simulink model "Raider_test"  (R2016a)
settings: Solver=VariableStepAuto  StartTime=0.0  StopTime=inf  RelTol=1e-3
model workspace (MAT data in the model file):
  SL_ROS_VariableLengthArrays_MaxSizes.CommonInfo.ArrayTruncateAction = 'EmitWarning'
  SL_ROS_VariableLengthArrays_MaxSizes.MsgTypeMap = containers.Map
  SL_ROS_VariableLengthArrays_MaxSizes.MsgTypeMap.serialization.keys = {'sensor_msgs/Image', 'sensor_msgs/JointState'}
  SL_ROS_VariableLengthArrays_MaxSizes.MsgTypeMap.serialization.values{1}(1).PropertyName = 'Encoding'
  SL_ROS_VariableLengthArrays_MaxSizes.MsgTypeMap.serialization.values{1}(1).DataType = 'uint8'
  SL_ROS_VariableLengthArrays_MaxSizes.MsgTypeMap.serialization.values{1}(1).MaxLength = 128
  SL_ROS_VariableLengthArrays_MaxSizes.MsgTypeMap.serialization.values{1}(2).PropertyName = 'Data'
  SL_ROS_VariableLengthArrays_MaxSizes.MsgTypeMap.serialization.values{1}(2).DataType = 'uint8'
  SL_ROS_VariableLengthArrays_MaxSizes.MsgTypeMap.serialization.values{1}(2).MaxLength = 2000000
  SL_ROS_VariableLengthArrays_MaxSizes.MsgTypeMap.serialization.values{2}(1).PropertyName = 'Name'
  SL_ROS_VariableLengthArrays_MaxSizes.MsgTypeMap.serialization.values{2}(1).DataType = 'std_msgs/String'
  SL_ROS_VariableLengthArrays_MaxSizes.MsgTypeMap.serialization.values{2}(1).MaxLength = 20
  SL_ROS_VariableLengthArrays_MaxSizes.MsgTypeMap.serialization.values{2}(2).PropertyName = 'Position'
  SL_ROS_VariableLengthArrays_MaxSizes.MsgTypeMap.serialization.values{2}(2).DataType = 'double'
  SL_ROS_VariableLengthArrays_MaxSizes.MsgTypeMap.serialization.values{2}(2).MaxLength = 128
  SL_ROS_VariableLengthArrays_MaxSizes.MsgTypeMap.serialization.values{2}(3).PropertyName = 'Velocity'
  SL_ROS_VariableLengthArrays_MaxSizes.MsgTypeMap.serialization.values{2}(3).DataType = 'double'
  SL_ROS_VariableLengthArrays_MaxSizes.MsgTypeMap.serialization.values{2}(3).MaxLength = 128
  SL_ROS_VariableLengthArrays_MaxSizes.MsgTypeMap.serialization.values{2}(4).PropertyName = 'Effort'
  SL_ROS_VariableLengthArrays_MaxSizes.MsgTypeMap.serialization.values{2}(4).DataType = 'double'
  SL_ROS_VariableLengthArrays_MaxSizes.MsgTypeMap.serialization.values{2}(4).MaxLength = 128
  SL_ROS_VariableLengthArrays_MaxSizes.MsgTypeMap.serialization.uniformity = 0
  SL_ROS_VariableLengthArrays_MaxSizes.MsgTypeMap.serialization.keyType = 'char'
  SL_ROS_VariableLengthArrays_MaxSizes.MsgTypeMap.serialization.valueType = 'any'
libraries: robotlib x81
settings Model: Creator=xavidz  LastModifiedBy=xavidz
settings DataIOCC: LimitDataPoints=on
settings DebuggingCC: AllowSymbolicDim=off
settings ModelReferenceCC: PropagateSignalLabelsOutOfModel=off
settings GRTTargetCC: GeneratePreprocessorConditionals=Use local settings

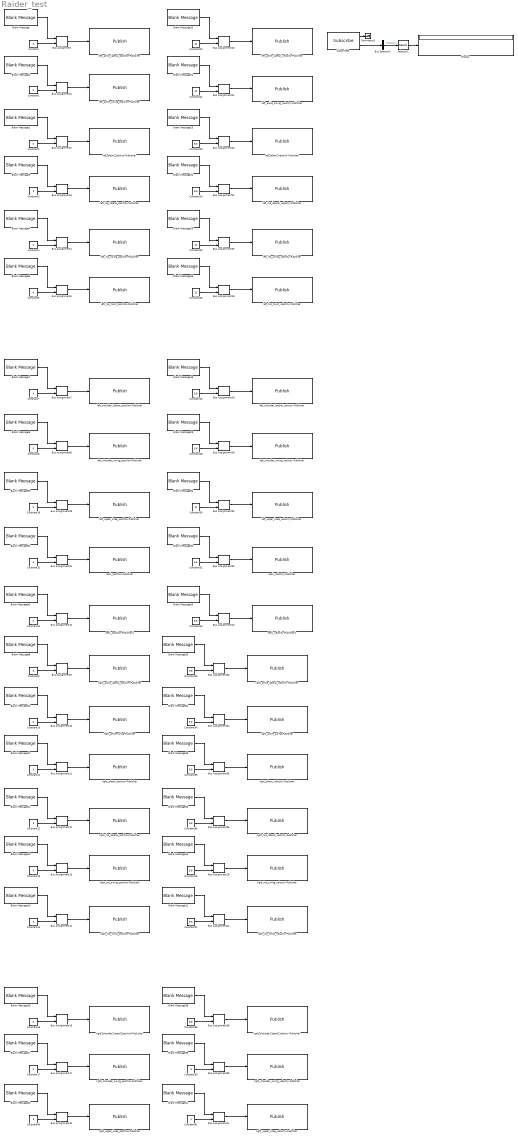
== system Raider_test ==
  Blank Message{,1..5,7..14,16..26,28..36,38..43} (40 alike) : robotlib/Blank Message  SourceLibraryInfo=This block requires Robotics System Toolbox  messageType=std_msgs/Float64  SampleTime=inf
  Bus Assignment{,1..5,7..14,16..26,28..36,38..43} (40 alike) : BusAssignment  AssignedSignals=Data
  Bus Selector3 : BusSelector  OutputSignals=Position
  Constant{,1..2,4..5,7..14,16..17,29,31,40,42} (19 alike) : Constant  Value=0
  Constant{18..19,21,23..24,28,32..36,38,43} (13 alike) : Constant  Value=5.6
  Constant{20,22,25..26,30} (5 alike) : Constant  Value=12
  Constant3 : Constant  Value=2
  Constant39 : Constant  Value=3
  Constant41 : Constant
  Display : Display
  Selector1 : Selector  IndexOptions=Select all  Indices=1  OutputSizes=1
  Subscribe3 : robotlib/Subscribe  SourceLibraryInfo=This block requires Robotics System Toolbox  topicSource=Select from ROS network  topic=/raider/joint_states  messageType=sensor_msgs/JointState  sampleTime=-1  messageQueueLength=1
  Terminator3 : Terminator
  left_ankle_lateral_position-Publisher : robotlib/Publish  SourceLibraryInfo=This block requires Robotics System Toolbox  topicSource=Select from ROS network  topic=/raider/l_ankle_lateral_position_controller/command  messageType=std_msgs/Float64  messageQueueLength=1
  left_ankle_lateral_velocity-Publisher : robotlib/Publish  SourceLibraryInfo=This block requires Robotics System Toolbox  topicSource=Select from ROS network  topic=/raider/l_ankle_lateral_velocity_controller/command  messageType=std_msgs/Float64  messageQueueLength=1
  left_ankle_swing_position-Publisher : robotlib/Publish  SourceLibraryInfo=This block requires Robotics System Toolbox  topicSource=Select from ROS network  topic=/raider/l_ankle_swing_position_controller/command  messageType=std_msgs/Float64  messageQueueLength=1
  left_ankle_swing_velocity-Publisher : robotlib/Publish  SourceLibraryInfo=This block requires Robotics System Toolbox  topicSource=Select from ROS network  topic=/raider/l_ankle_swing_velocity_controller/command  messageType=std_msgs/Float64  messageQueueLength=1
  left_elbow_position-Publisher : robotlib/Publish  SourceLibraryInfo=This block requires Robotics System Toolbox  topicSource=Select from ROS network  topic=/raider/l_elbow_position_controller/command  messageType=std_msgs/Float64  messageQueueLength=1
  left_elbow_velocity-Publisher : robotlib/Publish  SourceLibraryInfo=This block requires Robotics System Toolbox  topicSource=Select from ROS network  topic=/raider/l_elbow_velocity_controller/command  messageType=std_msgs/Float64  messageQueueLength=1
  left_hip_lateral_position-Publisher : robotlib/Publish  SourceLibraryInfo=This block requires Robotics System Toolbox  topicSource=Select from ROS network  topic=/raider/l_hip_lateral_position_controller/command  messageType=std_msgs/Float64  messageQueueLength=1
  left_hip_lateral_velocity-Publisher : robotlib/Publish  SourceLibraryInfo=This block requires Robotics System Toolbox  topicSource=Select from ROS network  topic=/raider/l_hip_lateral_velocity_controller/command  messageType=std_msgs/Float64  messageQueueLength=1
  left_hip_swing_position-Publisher : robotlib/Publish  SourceLibraryInfo=This block requires Robotics System Toolbox  topicSource=Select from ROS network  topic=/raider/l_hip_swing_position_controller/command  messageType=std_msgs/Float64  messageQueueLength=1
  left_hip_swing_velocity-Publisher : robotlib/Publish  SourceLibraryInfo=This block requires Robotics System Toolbox  topicSource=Select from ROS network  topic=/raider/l_hip_swing_velocity_controller/command  messageType=std_msgs/Float64  messageQueueLength=1
  left_hip_twist_position-Publisher : robotlib/Publish  SourceLibraryInfo=This block requires Robotics System Toolbox  topicSource=Select from ROS network  topic=/raider/l_hip_twist_position_controller/command  messageType=std_msgs/Float64  messageQueueLength=1
  left_hip_twist_velocity-Publisher : robotlib/Publish  SourceLibraryInfo=This block requires Robotics System Toolbox  topicSource=Select from ROS network  topic=/raider/l_hip_twist_velocity_controller/command  messageType=std_msgs/Float64  messageQueueLength=1
  left_shoulder_lateral_position-Publisher : robotlib/Publish  SourceLibraryInfo=This block requires Robotics System Toolbox  topicSource=Select from ROS network  topic=/raider/l_shoulder_lateral_position_controller/command  messageType=std_msgs/Float64  messageQueueLength=1
  left_shoulder_lateral_velocity-Publisher : robotlib/Publish  SourceLibraryInfo=This block requires Robotics System Toolbox  topicSource=Select from ROS network  topic=/raider/l_shoulder_lateral_velocity_controller/command  messageType=std_msgs/Float64  messageQueueLength=1
  left_shoulder_swing_position-Publisher : robotlib/Publish  SourceLibraryInfo=This block requires Robotics System Toolbox  topicSource=Select from ROS network  topic=/raider/l_shoulder_swing_position_controller/command  messageType=std_msgs/Float64  messageQueueLength=1
  left_shoulder_swing_velocity-Publisher : robotlib/Publish  SourceLibraryInfo=This block requires Robotics System Toolbox  topicSource=Select from ROS network  topic=/raider/l_shoulder_swing_velocity_controller/command  messageType=std_msgs/Float64  messageQueueLength=1
  left_upper_knee_position-Publisher : robotlib/Publish  SourceLibraryInfo=This block requires Robotics System Toolbox  topicSource=Select from ROS network  topic=/raider/l_upper_knee_position_controller/command  messageType=std_msgs/Float64  messageQueueLength=1
  left_upper_knee_velocity-Publisher : robotlib/Publish  SourceLibraryInfo=This block requires Robotics System Toolbox  topicSource=Select from ROS network  topic=/raider/l_upper_knee_velocity_controller/command  messageType=std_msgs/Float64  messageQueueLength=1
  neck_position-Publisher : robotlib/Publish  SourceLibraryInfo=This block requires Robotics System Toolbox  topicSource=Select from ROS network  topic=/raider/neck_position_controller/command  messageType=std_msgs/Float64  messageQueueLength=1
  neck_position-Publisher1 : robotlib/Publish  SourceLibraryInfo=This block requires Robotics System Toolbox  topicSource=Select from ROS network  topic=/raider/middle_hip_twist_position_controller/command  messageType=std_msgs/Float64  messageQueueLength=1
  neck_velocity-Publisher : robotlib/Publish  SourceLibraryInfo=This block requires Robotics System Toolbox  topicSource=Select from ROS network  topic=/raider/neck_velocity_controller/command  messageType=std_msgs/Float64  messageQueueLength=1
  neck_velocity-Publisher1 : robotlib/Publish  SourceLibraryInfo=This block requires Robotics System Toolbox  topicSource=Select from ROS network  topic=/raider/middle_hip_twist_velocity_controller/command  messageType=std_msgs/Float64  messageQueueLength=1
  right_ankle-swing-Publisher : robotlib/Publish  SourceLibraryInfo=This block requires Robotics System Toolbox  topicSource=Select from ROS network  topic=/raider/r_ankle_swing_position_controller/command  messageType=std_msgs/Float64  messageQueueLength=1
  right_ankle_lateral_position-Publisher : robotlib/Publish  SourceLibraryInfo=This block requires Robotics System Toolbox  topicSource=Select from ROS network  topic=/raider/r_ankle_lateral_position_controller/command  messageType=std_msgs/Float64  messageQueueLength=1
  right_ankle_lateral_velocity-Publisher : robotlib/Publish  SourceLibraryInfo=This block requires Robotics System Toolbox  topicSource=Select from ROS network  topic=/raider/r_ankle_lateral_velocity_controller/command  messageType=std_msgs/Float64  messageQueueLength=1
  right_ankle_swing-Publisher : robotlib/Publish  SourceLibraryInfo=This block requires Robotics System Toolbox  topicSource=Select from ROS network  topic=/raider/r_ankle_swing_velocity_controller/command  messageType=std_msgs/Float64  messageQueueLength=1
  right_elbow_position-Publisher : robotlib/Publish  SourceLibraryInfo=This block requires Robotics System Toolbox  topicSource=Select from ROS network  topic=/raider/r_elbow_position_controller/command  messageType=std_msgs/Float64  messageQueueLength=1
  right_elbow_velocity-Publisher : robotlib/Publish  SourceLibraryInfo=This block requires Robotics System Toolbox  topicSource=Select from ROS network  topic=/raider/r_elbow_velocity_controller/command  messageType=std_msgs/Float64  messageQueueLength=1
  right_hip_lateral_position-Publisher : robotlib/Publish  SourceLibraryInfo=This block requires Robotics System Toolbox  topicSource=Select from ROS network  topic=/raider/r_hip_lateral_position_controller/command  messageType=std_msgs/Float64  messageQueueLength=1
  right_hip_lateral_velocity-Publisher : robotlib/Publish  SourceLibraryInfo=This block requires Robotics System Toolbox  topicSource=Select from ROS network  topic=/raider/r_hip_lateral_velocity_controller/command  messageType=std_msgs/Float64  messageQueueLength=1
  right_hip_swing_position-Publisher : robotlib/Publish  SourceLibraryInfo=This block requires Robotics System Toolbox  topicSource=Select from ROS network  topic=/raider/r_hip_swing_position_controller/command  messageType=std_msgs/Float64  messageQueueLength=1
  right_hip_swing_velocity-Publisher : robotlib/Publish  SourceLibraryInfo=This block requires Robotics System Toolbox  topicSource=Select from ROS network  topic=/raider/r_hip_swing_velocity_controller/command  messageType=std_msgs/Float64  messageQueueLength=1
  right_hip_twist_position-Publisher : robotlib/Publish  SourceLibraryInfo=This block requires Robotics System Toolbox  topicSource=Select from ROS network  topic=/raider/r_hip_twist_position_controller/command  messageType=std_msgs/Float64  messageQueueLength=1
  right_hip_twist_velocity-Publisher : robotlib/Publish  SourceLibraryInfo=This block requires Robotics System Toolbox  topicSource=Select from ROS network  topic=/raider/r_hip_twist_velocity_controller/command  messageType=std_msgs/Float64  messageQueueLength=1
  right_shoulder_lateral_position-Publisher : robotlib/Publish  SourceLibraryInfo=This block requires Robotics System Toolbox  topicSource=Select from ROS network  topic=/raider/r_shoulder_lateral_position_controller/command  messageType=std_msgs/Float64  messageQueueLength=1
  right_shoulder_lateral_velocity-Publisher : robotlib/Publish  SourceLibraryInfo=This block requires Robotics System Toolbox  topicSource=Select from ROS network  topic=/raider/r_shoulder_lateral_velocity_controller/command  messageType=std_msgs/Float64  messageQueueLength=1
  right_shoulder_swing_position-Publisher : robotlib/Publish  SourceLibraryInfo=This block requires Robotics System Toolbox  topicSource=Select from ROS network  topic=/raider/r_shoulder_swing_position_controller/command  messageType=std_msgs/Float64  messageQueueLength=1
  right_shoulder_swing_velocity-Publisher : robotlib/Publish  SourceLibraryInfo=This block requires Robotics System Toolbox  topicSource=Select from ROS network  topic=/raider/r_shoulder_swing_velocity_controller/command  messageType=std_msgs/Float64  messageQueueLength=1
  right_upper_knee_position-Publisher : robotlib/Publish  SourceLibraryInfo=This block requires Robotics System Toolbox  topicSource=Select from ROS network  topic=/raider/r_upper_knee_position_controller/command  messageType=std_msgs/Float64  messageQueueLength=1
  right_upper_knee_velocity-Publisher : robotlib/Publish  SourceLibraryInfo=This block requires Robotics System Toolbox  topicSource=Select from ROS network  topic=/raider/r_upper_knee_velocity_controller/command  messageType=std_msgs/Float64  messageQueueLength=1
  wires:
  Blank Message/1 -> Bus Assignment/1
  Bus Assignment/1 -> left_ankle_lateral_position-Publisher/1
  Constant/1 -> Bus Assignment/2
  Blank Message1/1 -> Bus Assignment1/1
  Bus Assignment1/1 -> left_ankle_swing_position-Publisher/1
  Constant1/1 -> Bus Assignment1/2
  Blank Message2/1 -> Bus Assignment2/1
  Bus Assignment2/1 -> left_elbow_position-Publisher/1
  Constant2/1 -> Bus Assignment2/2
  Blank Message3/1 -> Bus Assignment3/1
  Bus Assignment3/1 -> left_hip_lateral_position-Publisher/1
  Constant3/1 -> Bus Assignment3/2
  Blank Message4/1 -> Bus Assignment4/1
  Bus Assignment4/1 -> left_hip_swing_position-Publisher/1
  Constant4/1 -> Bus Assignment4/2
  Blank Message5/1 -> Bus Assignment5/1
  Bus Assignment5/1 -> left_hip_twist_position-Publisher/1
  Constant5/1 -> Bus Assignment5/2
  Blank Message7/1 -> Bus Assignment7/1
  Bus Assignment7/1 -> left_shoulder_lateral_position-Publisher/1
  Constant7/1 -> Bus Assignment7/2
  Blank Message8/1 -> Bus Assignment8/1
  Bus Assignment8/1 -> left_shoulder_swing_position-Publisher/1
  Constant8/1 -> Bus Assignment8/2
  Blank Message9/1 -> Bus Assignment9/1
  Bus Assignment9/1 -> right_ankle_lateral_position-Publisher/1
  Constant9/1 -> Bus Assignment9/2
  Blank Message10/1 -> Bus Assignment10/1
  Bus Assignment10/1 -> right_ankle-swing-Publisher/1
  Constant10/1 -> Bus Assignment10/2
  Blank Message11/1 -> Bus Assignment11/1
  Bus Assignment11/1 -> right_elbow_position-Publisher/1
  Constant11/1 -> Bus Assignment11/2
  Blank Message12/1 -> Bus Assignment12/1
  Bus Assignment12/1 -> right_hip_lateral_position-Publisher/1
  Constant12/1 -> Bus Assignment12/2
  Blank Message13/1 -> Bus Assignment13/1
  Bus Assignment13/1 -> right_hip_swing_position-Publisher/1
  Constant13/1 -> Bus Assignment13/2
  Blank Message14/1 -> Bus Assignment14/1
  Bus Assignment14/1 -> right_hip_twist_position-Publisher/1
  Constant14/1 -> Bus Assignment14/2
  Blank Message16/1 -> Bus Assignment16/1
  Bus Assignment16/1 -> right_shoulder_lateral_position-Publisher/1
  Constant16/1 -> Bus Assignment16/2
  Blank Message17/1 -> Bus Assignment17/1
  Bus Assignment17/1 -> right_shoulder_swing_position-Publisher/1
  Constant17/1 -> Bus Assignment17/2
  Blank Message21/1 -> Bus Assignment21/1
  Bus Assignment21/1 -> right_hip_twist_velocity-Publisher/1
  Constant21/1 -> Bus Assignment21/2
  Blank Message18/1 -> Bus Assignment18/1
  Bus Assignment18/1 -> right_hip_swing_velocity-Publisher/1
  Constant18/1 -> Bus Assignment18/2
  Blank Message19/1 -> Bus Assignment19/1
  Bus Assignment19/1 -> left_shoulder_lateral_velocity-Publisher/1
  Constant19/1 -> Bus Assignment19/2
  Blank Message20/1 -> Bus Assignment20/1
  Bus Assignment20/1 -> left_ankle_lateral_velocity-Publisher/1
  Constant20/1 -> Bus Assignment20/2
  Subscribe3/1 -> Terminator3/1
  Subscribe3/2 -> Bus Selector3/1
  Blank Message22/1 -> Bus Assignment22/1
  Bus Assignment22/1 -> left_ankle_swing_velocity-Publisher/1
  Constant22/1 -> Bus Assignment22/2
  Blank Message23/1 -> Bus Assignment23/1
  Bus Assignment23/1 -> left_elbow_velocity-Publisher/1
  Constant23/1 -> Bus Assignment23/2
  Blank Message24/1 -> Bus Assignment24/1
  Bus Assignment24/1 -> left_hip_lateral_velocity-Publisher/1
  Constant24/1 -> Bus Assignment24/2
  Blank Message25/1 -> Bus Assignment25/1
  Bus Assignment25/1 -> left_hip_swing_velocity-Publisher/1
  Constant25/1 -> Bus Assignment25/2
  Blank Message26/1 -> Bus Assignment26/1
  Bus Assignment26/1 -> left_hip_twist_velocity-Publisher/1
  Constant26/1 -> Bus Assignment26/2
  Blank Message28/1 -> Bus Assignment28/1
  Bus Assignment28/1 -> left_shoulder_swing_velocity-Publisher/1
  Constant28/1 -> Bus Assignment28/2
  Blank Message29/1 -> Bus Assignment29/1
  Bus Assignment29/1 -> left_upper_knee_position-Publisher/1
  Constant29/1 -> Bus Assignment29/2
  Blank Message30/1 -> Bus Assignment30/1
  Bus Assignment30/1 -> left_upper_knee_velocity-Publisher/1
  Constant30/1 -> Bus Assignment30/2
  Blank Message31/1 -> Bus Assignment31/1
  Bus Assignment31/1 -> neck_position-Publisher/1
  Constant31/1 -> Bus Assignment31/2
  Blank Message32/1 -> Bus Assignment32/1
  Bus Assignment32/1 -> neck_velocity-Publisher/1
  Constant32/1 -> Bus Assignment32/2
  Blank Message33/1 -> Bus Assignment33/1
  Bus Assignment33/1 -> right_ankle_lateral_velocity-Publisher/1
  Constant33/1 -> Bus Assignment33/2
  Blank Message34/1 -> Bus Assignment34/1
  Bus Assignment34/1 -> right_ankle_swing-Publisher/1
  Constant34/1 -> Bus Assignment34/2
  Blank Message35/1 -> Bus Assignment35/1
  Bus Assignment35/1 -> right_elbow_velocity-Publisher/1
  Constant35/1 -> Bus Assignment35/2
  Blank Message36/1 -> Bus Assignment36/1
  Bus Assignment36/1 -> right_hip_lateral_velocity-Publisher/1
  Constant36/1 -> Bus Assignment36/2
  Blank Message38/1 -> Bus Assignment38/1
  Bus Assignment38/1 -> right_shoulder_lateral_velocity-Publisher/1
  Constant38/1 -> Bus Assignment38/2
  Blank Message39/1 -> Bus Assignment39/1
  Bus Assignment39/1 -> right_shoulder_swing_velocity-Publisher/1
  Constant39/1 -> Bus Assignment39/2
  Blank Message40/1 -> Bus Assignment40/1
  Bus Assignment40/1 -> right_upper_knee_position-Publisher/1
  Constant40/1 -> Bus Assignment40/2
  Blank Message41/1 -> Bus Assignment41/1
  Bus Assignment41/1 -> right_upper_knee_velocity-Publisher/1
  Constant41/1 -> Bus Assignment41/2
  Blank Message42/1 -> Bus Assignment42/1
  Bus Assignment42/1 -> neck_position-Publisher1/1
  Constant42/1 -> Bus Assignment42/2
  Blank Message43/1 -> Bus Assignment43/1
  Bus Assignment43/1 -> neck_velocity-Publisher1/1
  Constant43/1 -> Bus Assignment43/2
  Bus Selector3/1 -> Selector1/1  "<Position>"
  Selector1/1 -> Display/1
